simulink model "AVoWk3Prob3"  (R2021b)
settings: Solver=FixedStepAuto  StartTime=0.0  StopTime=10  FixedStep=.01  RelTol=1e-3  EnableMultiTasking=on
values from neighbouring files (symbols this model uses):
  a = 2    [AndyVoLab2.m]    (also in ME4391L_LAB2_Goulenko_P2.m)
  b = 3    [AndyVoLab2.m]    (also in ME4391L_LAB2_Goulenko_P2.m)
  c = 0.25    [AndyVoLab2.m]    (also in ME4391L_LAB2_Goulenko_P2.m)
  d = 1 * 2*pi    (= 6.28318530718)    [AndyVoLab2.m]    (also in ME4391L_LAB2_Goulenko_P2.m)
settings Model: ExtModeTrigDuration=10000  Creator=andyvo  LastModifiedBy=andyvo
settings SolverCC: AlgebraicLoopSolver=TrustRegion  PositivePriorityOrder=on
settings DataIOCC: ReturnWorkspaceOutputs=off
settings DebuggingCC: SFMachineParentedDataDiag=warning  ArithmeticOperatorsInVariantConditions=warning
settings SFSimCC: SimUseLocalCustomCode=off  CustomCodeUndefinedFunction=UseInterfaceOnly
settings RTWCC: Description=QUARC Win64 Target Using Toolchain  SystemTargetFile=quarc_win64.tlc  TemplateMakefile=quarc_default_tmf  RTWUseLocalCustomCode=off  Toolchain=QUARC win64 | nmake (64-bit Windows)  BuildConfiguration=Faster Runs
settings CodeAppCC: StateflowObjectComments=on
settings STFCustomTargetCC: TargetLangStandard=C99 (ISO)  ConcurrentExecutionCompliant=on  UseToolchainInfoCompliant=on  SystemTargetFile=quarc_win64.tlc
settings GRTTargetCC: ParMdlRefBuildCompliant=off  CompOptLevelCompliant=off  CombineOutputUpdateFcns=off  MatFileLogging=off  CPPClassGenCompliant=off  GRTInterface=on  ExtMode=on  ExtModeMexFile=quarc_comm
settings ConfigComp: CovMetricSettings=dswe

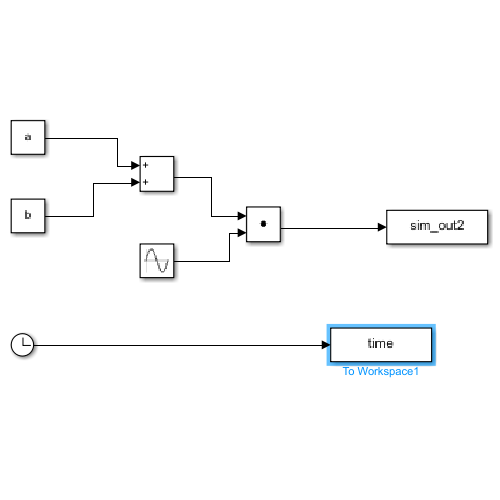
[thumbnail: Simulink's stored preview of the top-level diagram]
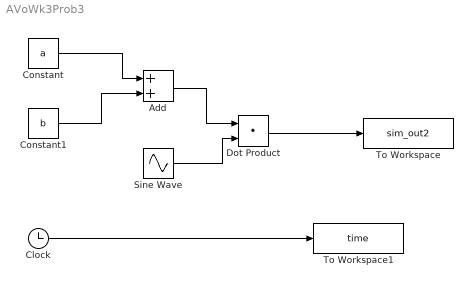
== system AVoWk3Prob3 ==
  Add : Sum
  Clock : Clock
  Constant : Constant  Value=a
  Constant1 : Constant  Value=b
  Dot Product : DotProduct  InputSameDT=on  OutDataTypeStr=Inherit: Inherit via internal rule
  Sine Wave : Sin  Amplitude=c  Frequency=d  SampleTime=0
  To Workspace : ToWorkspace  VariableName=sim_out2  SampleTime=-1
  To Workspace1 : ToWorkspace  VariableName=time  SampleTime=-1
  wires:
  Clock/1 -> To Workspace1/1
  Sine Wave/1 -> Dot Product/2
  Constant1/1 -> Add/2
  Add/1 -> Dot Product/1
  Constant/1 -> Add/1
  Dot Product/1 -> To Workspace/1
